simulink model "magnetometer_processing_test"  (R2016b)
settings: Solver=VariableStepAuto  StartTime=0.0  StopTime=100  RelTol=1e-3
values from neighbouring files (symbols this model uses):
  fsw_params = init_fsw_params()    [magnetometer_processing_test_init.m]
libraries: simulink x3, GPS_time_lib x1, aerolibtransform2 x1, mag_vec_lib x1, sensor_processing_libs x1, magnetometer_lib x1, time_coord_rotation_lib x1, tle2eci_coarse_lib x1
settings Model: Creator=Sean  LastModifiedBy=Sean

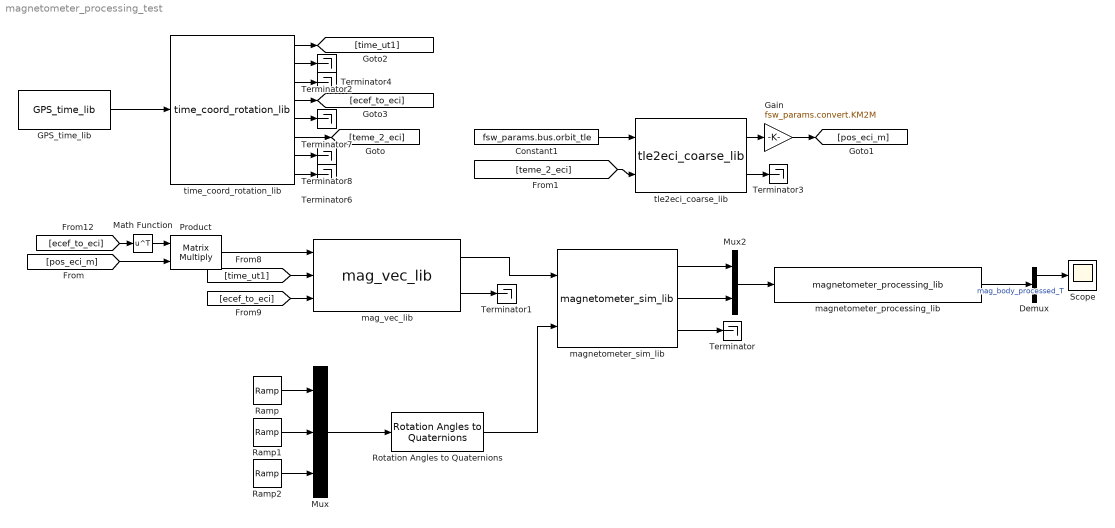
== system magnetometer_processing_test ==
  Constant1 : Constant  Value=fsw_params.bus.orbit_tle
  Demux : Demux  Outputs=[3 1]
  GPS_time_lib : GPS_time_lib/GPS_time_lib
  Gain : Gain  Gain=fsw_params.convert.KM2M
  Math Function : Math  Operator=transpose  SaturateOnIntegerOverflow=on
  Mux : Mux  Inputs=3
  Mux2 : Mux  Inputs=[3 1]
  Product : Product  Multiplication=Matrix(*)
  Ramp : simulink/Sources/Ramp  slope=1  start=0  X0=0
  Ramp1 : simulink/Sources/Ramp  slope=0  start=0  X0=0
  Ramp2 : simulink/Sources/Ramp  slope=0  start=0  X0=0
  Rotation Angles to Quaternions : aerolibtransform2/Rotation Angles to Quaternions  rotationOrder=ZYX
  Scope : Scope
  Terminator{,1..4,6..8} (8 alike) : Terminator
  mag_vec_lib : mag_vec_lib/mag_vec_lib
  magnetometer_processing_lib : sensor_processing_libs/magnetometer_processing_lib
  magnetometer_sim_lib : magnetometer_lib/magnetometer_sim_lib
  time_coord_rotation_lib : time_coord_rotation_lib/time_coord_rotation_lib
  tle2eci_coarse_lib : tle2eci_coarse_lib/tle2eci_coarse_lib
  wires:
  magnetometer_sim_lib/2 -> Mux2/2
  magnetometer_sim_lib/1 -> Mux2/1
  Mux2/1 -> magnetometer_processing_lib/1
  magnetometer_sim_lib/3 -> Terminator/1
  [time_ut1] -> mag_vec_lib/2
  [pos_eci_m] -> Product/2
  Product/1 -> mag_vec_lib/1
  mag_vec_lib/2 -> Terminator1/1
  mag_vec_lib/1 -> magnetometer_sim_lib/1
  [ecef_to_eci] -> mag_vec_lib/3
  [ecef_to_eci] -> Math Function/1
  Math Function/1 -> Product/1
  Constant1/1 -> tle2eci_coarse_lib/1
  tle2eci_coarse_lib/1 -> Gain/1
  tle2eci_coarse_lib/2 -> Terminator3/1
  Gain/1 -> [pos_eci_m]
  Rotation Angles to Quaternions/1 -> magnetometer_sim_lib/2
  time_coord_rotation_lib/5 -> Terminator7/1
  time_coord_rotation_lib/8 -> Terminator6/1
  time_coord_rotation_lib/6 -> [teme_2_eci]
  time_coord_rotation_lib/3 -> Terminator4/1
  GPS_time_lib/1 -> time_coord_rotation_lib/1
  time_coord_rotation_lib/4 -> [ecef_to_eci]
  time_coord_rotation_lib/2 -> Terminator2/1
  time_coord_rotation_lib/7 -> Terminator8/1
  time_coord_rotation_lib/1 -> [time_ut1]
  magnetometer_processing_lib/1 -> Demux/1  "mag_body_processed_T"
  [teme_2_eci] -> tle2eci_coarse_lib/2
  Demux/1 -> Scope/1
  Ramp1/1 -> Mux/2
  Ramp/1 -> Mux/1
  Ramp2/1 -> Mux/3
  Mux/1 -> Rotation Angles to Quaternions/1
